simulink model "Dc_machine_modelling"  (R2016a)
settings: Solver=VariableStepAuto  StartTime=0.0  StopTime=20  RelTol=1e-3
libraries: powerlib x18, simulink x1
settings Model: Creator=AT Once  LastModifiedBy=AT Once

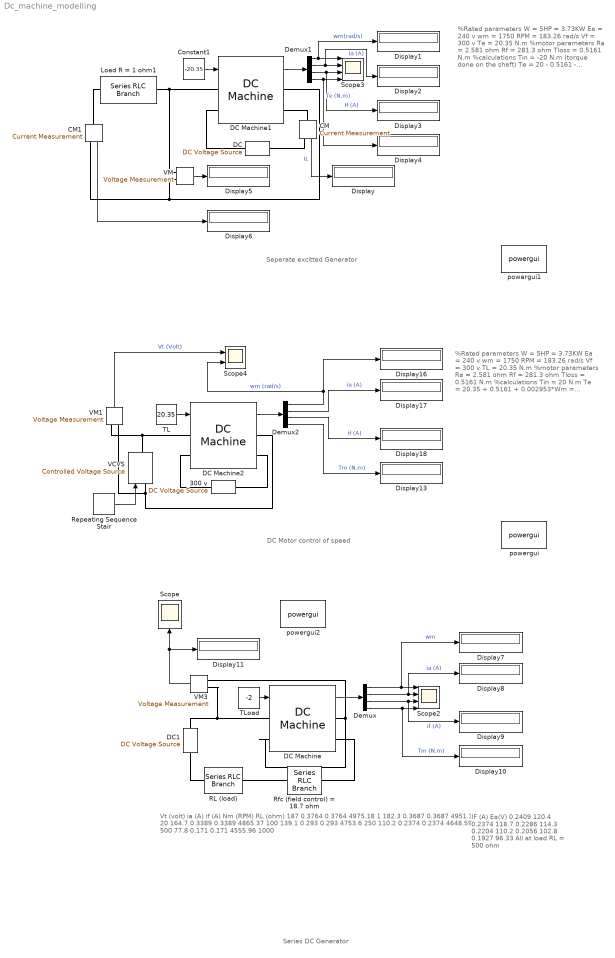
== system Dc_machine_modelling ==
  note: Series DC Generator
  note: Vt (volt)
      | ia (A)
      | if (A)
      | Nm (RPM)
      | RL (ohm)
      |
      | 187
      | 0.3764
      | 0.3764
      | 4975.18
      | 1
      |
      | 182.3
      | 0.3687
      | 0.3687
      | 4951.3
      | 20
      |
      | 164.7
      | 0.3389
      | 0.3389
      | 4865.37
      | 100
      |
      | 139.1
      | 0.293
      | 0.293
      | 4753.6
      | 250
      |
      | 110.2
      | 0.2374
      | 0.2374
      | 4648.59
      | 500
      |
      | 77.8
      | 0.171
      | 0.171
      | 4555.96
      | 1000
  note: DC Motor control of speed
  note: Seperate excitted Generator
  note: IF (A)
      | Ea(V)
      |
      | 0.2409
      | 120.4
      |
      | 0.2374
      | 118.7
      |
      | 0.2286
      | 114.3
      |
      | 0.2204
      | 110.2
      |
      | 0.2056
      | 102.8
      |
      | 0.1927
      | 96.33
      |
      | All at load
      | RL = 500 ohm
  note: %Rated parameters
      | W = 5HP = 3.73KW
      | Ea = 240 v
      | wm = 1750 RPM = 183.26 rad/s
      | Vf = 300 v
      | Te = 20.35 N.m
      |
      | %motor parameters
      | Ra = 2.581 ohm
      | Rf = 281.3 ohm
      | Tloss = 0.5161 N.m
      |
      | %calculations
      | Tin = -20 N.m (torque done on the shaft)
      | Te = 20 - 0.5161 - 0.002953*Wm = N.m
  note: %Rated parameters
      | W = 5HP = 3.73KW
      | Ea = 240 v
      | wm = 1750 RPM = 183.26 rad/s
      | Vf = 300 v
      | TL = 20.35 N.m
      |
      | %motor parameters
      | Ra = 2.581 ohm
      | Rf = 281.3 ohm
      | Tloss = 0.5161 N.m
      |
      | %calculations
      | Tin = 20 N.m
      | Te = 20.35 + 0.5161 + 0.002953*Wm =
      | 21.407 N.m
  300 v : powerlib/Electrical Sources/DC Voltage Source  Amplitude=300  Measurements=None
  CM : powerlib/Measurements/Current Measurement  PhasorSimulation=off  OutputType=Complex  PSBequivalent=0
  CM1 : powerlib/Measurements/Current Measurement  PhasorSimulation=off  OutputType=Complex  PSBequivalent=0
  Constant1 : Constant  Value=-20.35
  DC : powerlib/Electrical Sources/DC Voltage Source  Amplitude=150  Measurements=None
  DC Machine : powerlib/Machines/DC Machine  PresetModel=01: 5HP 240V 1750RPM Field:300V  MechanicalLoad=Torque TL  FieldType=Wound  ShowDetailedParameters=on  MeasurementBus=off  RLa=[2.581 0.028]  RLf=[281.3 156]  Laf=0.9483  MachineConstant=Torque constant (N.m/A)  Ke=1.8  Kt=1.8  J=0.02215  Bm=0.002953  Tf=0.5161  w0=1  Ifinit=10  TsPowergui=0  TsBlock=-1
  DC Machine1 : powerlib/Machines/DC Machine  PresetModel=01: 5HP 240V 1750RPM Field:300V  MechanicalLoad=Torque TL  FieldType=Wound  ShowDetailedParameters=on  MeasurementBus=off  RLa=[2.581 0.028]  RLf=[281.3 156]  Laf=0.9483  MachineConstant=Torque constant (N.m/A)  Ke=1.8  Kt=1.8  J=0.02215  Bm=0.002953  Tf=0.5161  w0=0  Ifinit=0  TsPowergui=0  TsBlock=-1
  DC Machine2 : powerlib/Machines/DC Machine  PresetModel=01: 5HP 240V 1750RPM Field:300V  MechanicalLoad=Torque TL  FieldType=Wound  ShowDetailedParameters=on  MeasurementBus=off  RLa=[2.581 0.028]  RLf=[281.3 156]  Laf=0.9483  MachineConstant=Torque constant (N.m/A)  Ke=1.8  Kt=1.8  J=0.02215  Bm=0.002953  Tf=0.5161  w0=0  Ifinit=0  TsPowergui=0  TsBlock=-1
  DC1 : powerlib/Electrical Sources/DC Voltage Source  Amplitude=300  Measurements=None
  Demux : Demux
  Demux1 : Demux
  Demux2 : Demux
  Display{,1..11,13,16..18} (16 alike) : Display
  Load R = 1 ohm1 : powerlib/Elements/Series RLC Branch  LConnTagsString=__new0  RConnTagsString=__new0  BranchType=R  Resistance=1  Inductance=1e-3  SetiL0=off  InitialCurrent=0  Capacitance=1e-6  Setx0=off  InitialVoltage=0  Measurements=None
  "RL (load) " : powerlib/Elements/Series RLC Branch  LConnTagsString=__new0  RConnTagsString=__new0  BranchType=R  Resistance=1000  Inductance=1e-3  SetiL0=off  InitialCurrent=0  Capacitance=1e-6  Setx0=off  InitialVoltage=0  Measurements=None
  Repeating Sequence Stair : simulink/Sources/Repeating Sequence Stair  OutValues=[0 80 160 240].'  tsamp=10  OutMin=[]  OutMax=[]  OutDataTypeStr=double  OutputDataTypeScalingMode=double  OutDataType=fixdt(0,8)  ConRadixGroup=Best Precision: Vector-wise  OutScaling=2^-12
  Rfc (field control) = 18.7 ohm : powerlib/Elements/Series RLC Branch  LConnTagsString=__new0  RConnTagsString=__new0  BranchType=R  Resistance=18.7  Inductance=1e-3  SetiL0=off  InitialCurrent=0  Capacitance=1e-6  Setx0=off  InitialVoltage=0  Measurements=None
  Scope : Scope
  Scope2 : Scope  NumInputPorts=4
  Scope3 : Scope  NumInputPorts=4
  Scope4 : Scope  NumInputPorts=2
  TL : Constant  Value=20.35
  TLoad : Constant  Value=-2
  VCVS : powerlib/Electrical Sources/Controlled Voltage Source  Initialize=on  Source_Type=AC  Amplitude=0  Phase=0  Frequency=0  Measurements=None
  VM : powerlib/Measurements/Voltage Measurement  PhasorSimulation=off  OutputType=Complex  PSBequivalent=0
  VM1 : powerlib/Measurements/Voltage Measurement  PhasorSimulation=off  OutputType=Complex  PSBequivalent=0
  VM3 : powerlib/Measurements/Voltage Measurement  PhasorSimulation=off  OutputType=Complex  PSBequivalent=0
  powergui : powerlib/powergui  Priority=1  SimulationMode=Discrete  SolverType=Tustin/Backward Euler (TBE)  SampleTime=50e-6  frequency=60  SPID=off  DisableSnubberDevices=off  DisableRonSwitches=off  DisableVfSwitches=off  SwTol=0  DisplayEquations=off  Interpol=off  ExternalGateDelay=off  methode=off  Ts=10  FunctionMessages=off  echomessages=off  HookPort=off  EnableUseOfTLC=off  x0status=blocks  frequencyindice=0  Pbase=100e6  ErrMax=1e-4  Iterations=50  UnitsV=kV  UnitsW=MW  buscounter=0  RestoreLinks=warning  ResistiveCurrentMeasurement=off  Frange=[0:2:500]  Ylog=off  Xlog=on  ShowGrid=off  save=off  variable=ZData  structure=0  ZoomFFT=off  StartTime=0.0  cycles=1  DisplayStyle=1  fundamental=60  FreqAxis=off  MaxFrequency=1000  frequencyindicesteady=1  RmsSteady=1  display=off
  powergui1 : powerlib/powergui  Priority=1  SimulationMode=Continuous  SolverType=Tustin/Backward Euler (TBE)  SampleTime=50e-6  frequency=60  SPID=off  DisableSnubberDevices=off  DisableRonSwitches=off  DisableVfSwitches=off  SwTol=0  DisplayEquations=off  Interpol=off  ExternalGateDelay=off  methode=off  Ts=10  FunctionMessages=off  echomessages=off  HookPort=off  EnableUseOfTLC=off  x0status=blocks  frequencyindice=0  Pbase=100e6  ErrMax=1e-4  Iterations=50  UnitsV=kV  UnitsW=MW  buscounter=0  RestoreLinks=warning  ResistiveCurrentMeasurement=off  Frange=[0:2:500]  Ylog=off  Xlog=on  ShowGrid=off  save=off  variable=ZData  structure=0  ZoomFFT=off  StartTime=0.0  cycles=1  DisplayStyle=1  fundamental=60  FreqAxis=off  MaxFrequency=1000  frequencyindicesteady=1  RmsSteady=1  display=off
  powergui2 : powerlib/powergui  Priority=1  SimulationMode=Continuous  SolverType=Tustin/Backward Euler (TBE)  SampleTime=50e-6  frequency=60  SPID=off  DisableSnubberDevices=off  DisableRonSwitches=off  DisableVfSwitches=off  SwTol=0  DisplayEquations=off  Interpol=off  ExternalGateDelay=off  methode=off  Ts=10  FunctionMessages=off  echomessages=off  HookPort=off  EnableUseOfTLC=off  x0status=blocks  frequencyindice=0  Pbase=100e6  ErrMax=1e-4  Iterations=50  UnitsV=kV  UnitsW=MW  buscounter=0  RestoreLinks=warning  ResistiveCurrentMeasurement=off  Frange=[0:2:500]  Ylog=off  Xlog=on  ShowGrid=off  save=off  variable=ZData  structure=0  ZoomFFT=off  StartTime=0.0  cycles=1  DisplayStyle=1  fundamental=60  FreqAxis=off  MaxFrequency=1000  frequencyindicesteady=1  RmsSteady=1  display=off
  wires:
  DC Machine/1 -> Demux/1
  Demux/1 -> Display7/1, Scope2/1  "wm"
  Demux/2 -> Display8/1, Scope2/2  "ia (A)"
  Demux/3 -> Display9/1, Scope2/3  "if (A)"
  Demux/4 -> Display10/1, Scope2/4  "Tm (N.m)"
  Constant1/1 -> DC Machine1/1
  Demux1/1 -> Display1/1, Scope3/1  "wm(rad/s)"
  Demux1/2 -> Display2/1, Scope3/2  "Ia (A)"
  Demux1/3 -> Display3/1, Scope3/3  "If (A)"
  Demux1/4 -> Display4/1, Scope3/4  "Te (N.m)"
  DC Machine1/1 -> Demux1/1
  CM/1 -> Display/1  "IL"
  VM/1 -> Display5/1
  CM1/1 -> Display6/1
  DC Machine2/1 -> Demux2/1
  Demux2/1 -> Scope4/2, Display16/1  "wm (rad/s)"
  Demux2/2 -> Display17/1  "ia (A)"
  Demux2/3 -> Display18/1  "if (A)"
  Demux2/4 -> Display13/1  "Tm (N.m)"
  TL/1 -> DC Machine2/1
  VM1/1 -> Scope4/1  "Vt (Volt)"
  Repeating Sequence Stair/1 -> VCVS/1
  TLoad/1 -> DC Machine/1
  VM3/1 -> Scope/1, Display11/1
  connections:
  DC/RConn1 -- DC Machine1/LConn2
  CM/LConn1 -- DC Machine1/RConn2
  CM/RConn1 -- DC/LConn1
  Load R = 1 ohm1/RConn1 -- VM/LConn1 -- DC Machine1/LConn1
  VM/LConn2 -- CM1/RConn1 -- DC Machine1/RConn1
  CM1/LConn1 -- Load R = 1 ohm1/LConn1
  DC Machine2/LConn2 -- 300 v/RConn1
  300 v/LConn1 -- DC Machine2/RConn2
  DC Machine2/LConn1 -- VCVS/RConn1 -- VM1/LConn1
  DC Machine2/RConn1 -- VM1/LConn2 -- VCVS/LConn1
  DC Machine/LConn2 -- VM3/LConn1 -- DC Machine/RConn1
  Rfc (field control) = 18.7 ohm/LConn1 -- "RL (load) "/RConn1
  DC1/LConn1 -- VM3/LConn2 -- DC Machine/LConn1
  DC1/RConn1 -- "RL (load) "/LConn1
  Rfc (field control) = 18.7 ohm/RConn1 -- DC Machine/RConn2
